simulink model "Lecture6Exercise"  (R2020b)
settings: Solver=VariableStepAuto  StartTime=0.0  StopTime=10.0  RelTol=1e-3
values from neighbouring files (symbols this model uses):
  Ad = [0.8, -0.36; 0.09, 0.98]    [Lecture4Exercise.m]
  Bd = [0.09; 0.0047]    [Lecture4Exercise.m]
  Cd = [0, 10]    [Lecture4Exercise.m]    (also in Lecture5Exercises.m = C; Lecture6Exercise.m = C)
  Ts = 1.5    [Lecture3Exercise.m]    (also in Lecture4Exercise.m = 6; Lecture5Exercises.m = 0.02; Lecture6Exercise.m = 1/fs)
undefined symbols (not defined in the file or in its folder): K_a, K_b, K_c
settings Model: Creator=sebastian  LastModifiedBy=sebastian

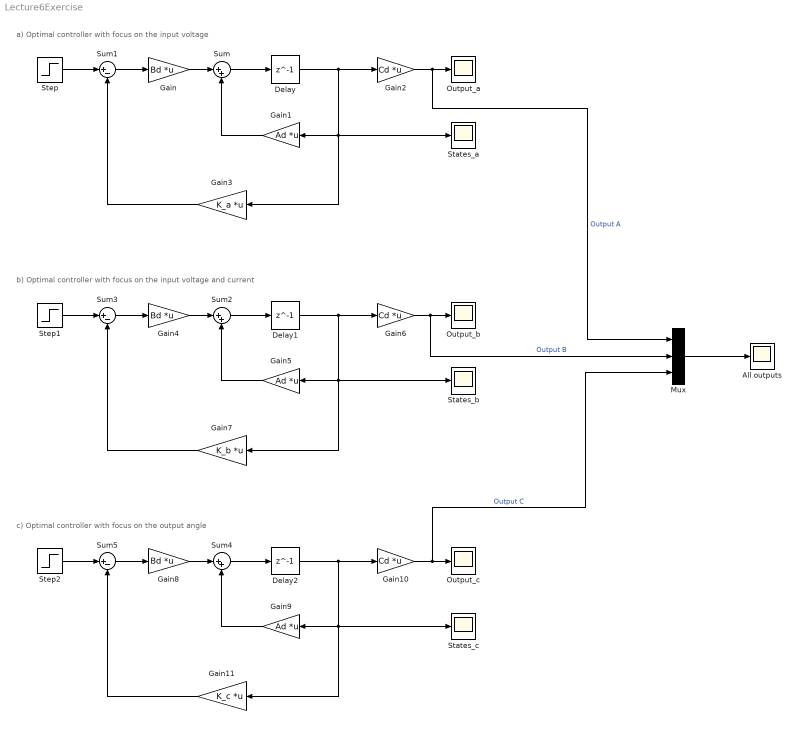
== system Lecture6Exercise ==
  note: a) Optimal controller with focus on the input voltage
  note: b) Optimal controller with focus on the input voltage and current
  note: c) Optimal controller with focus on the output angle
  All outputs : Scope
  Delay : Delay  DelayLength=1  SampleTime=Ts
  Delay1 : Delay  DelayLength=1  SampleTime=Ts
  Delay2 : Delay  DelayLength=1  SampleTime=Ts
  Gain : Gain  Gain=Bd  Multiplication=Matrix(K*u)
  Gain1 : Gain  Gain=Ad  Multiplication=Matrix(K*u)
  Gain10 : Gain  Gain=Cd  Multiplication=Matrix(K*u)
  Gain11 : Gain  Gain=K_c  Multiplication=Matrix(K*u)
  Gain2 : Gain  Gain=Cd  Multiplication=Matrix(K*u)
  Gain3 : Gain  Gain=K_a  Multiplication=Matrix(K*u)
  Gain4 : Gain  Gain=Bd  Multiplication=Matrix(K*u)
  Gain5 : Gain  Gain=Ad  Multiplication=Matrix(K*u)
  Gain6 : Gain  Gain=Cd  Multiplication=Matrix(K*u)
  Gain7 : Gain  Gain=K_b  Multiplication=Matrix(K*u)
  Gain8 : Gain  Gain=Bd  Multiplication=Matrix(K*u)
  Gain9 : Gain  Gain=Ad  Multiplication=Matrix(K*u)
  Mux : Mux  Inputs=3
  Output_a : Scope
  Output_b : Scope
  Output_c : Scope
  States_a : Scope
  States_b : Scope
  States_c : Scope
  Step : Step  SampleTime=0
  Step1 : Step  SampleTime=0
  Step2 : Step  SampleTime=0
  Sum : Sum  Inputs=|++
  Sum1 : Sum  Inputs=|+-
  Sum2 : Sum  Inputs=|++
  Sum3 : Sum  Inputs=|+-
  Sum4 : Sum  Inputs=|++
  Sum5 : Sum  Inputs=|+-
  wires:
  Gain/1 -> Sum/1
  Delay/1 -> Gain2/1, Gain3/1, States_a/1, Gain1/1
  Gain1/1 -> Sum/2
  Sum/1 -> Delay/1
  Step/1 -> Sum1/1
  Sum1/1 -> Gain/1
  Gain3/1 -> Sum1/2
  Gain2/1 -> Mux/1, Output_a/1  "Output A"
  Gain7/1 -> Sum3/2
  Sum3/1 -> Gain4/1
  Gain5/1 -> Sum2/2
  Delay1/1 -> Gain6/1, Gain7/1, States_b/1, Gain5/1
  Step1/1 -> Sum3/1
  Sum2/1 -> Delay1/1
  Gain6/1 -> Output_b/1, Mux/2  "Output B"
  Gain4/1 -> Sum2/1
  Gain11/1 -> Sum5/2
  Sum5/1 -> Gain8/1
  Gain9/1 -> Sum4/2
  Delay2/1 -> Gain10/1, Gain11/1, States_c/1, Gain9/1
  Step2/1 -> Sum5/1
  Sum4/1 -> Delay2/1
  Gain10/1 -> Mux/3, Output_c/1  "Output C"
  Gain8/1 -> Sum4/1
  Mux/1 -> All outputs/1
